simulink model "model_pompy"  (R2015a)
settings: Solver=ode4  StartTime=0.0  StopTime=34  FixedStep=0.01  RelTol=1e-3
values from neighbouring files (symbols this model uses):
  p1 = polyfit(PWM_level, pred_napelniania, 3)    [chka_pompy.m]    (also in chka_zawor_gora.m; modelPompaZawor.m)
settings Model: Creator=konra  LastModifiedBy=konra
settings DataIOCC: LimitDataPoints=off

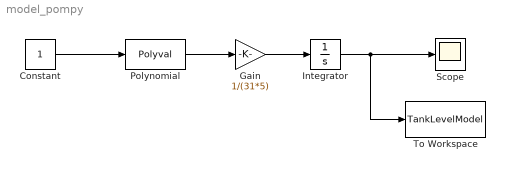
== system model_pompy ==
  Constant : Constant
  Gain : Gain  Gain=1/(31*5)
  Integrator : Integrator  InitialCondition=1.01
  Polynomial : Polyval  Coefs=p1
  Scope : Scope
  To Workspace : ToWorkspace  VariableName=TankLevelModel  SaveFormat=Structure With Time  SampleTime=-1
  wires:
  Gain/1 -> Integrator/1
  Integrator/1 -> To Workspace/1, Scope/1
  Constant/1 -> Polynomial/1
  Polynomial/1 -> Gain/1
